simulink model "Model"  (R2019a)
settings: Solver=ode45  StartTime=0.0  StopTime=10  MaxStep=1e-3  RelTol=1e-3  EnableMultiTasking=on
values from neighbouring files (symbols this model uses):
  Cpf1 = tf(1,[1/1.05,1])    [mainProjetCADV_2a.m]
  dPHRTrim = trimVal(1)    [mainProjetCADV_2a.m]
  dthrIdle = 0.1    [mainProjetCADV_2a.m]
  H = -inv(Ccm*inv(Acm-Bcm*Kcm)*Bcm)    [mainProjetCADV_2a.m]
  idelevator = 3    [mainProjetCADV_2a.m]
  KTS2MS = 1852 / 3600    (= 0.514444444444)    [mainProjetCADV_2a.m]
  thetaTrim = trimVal(3)    [mainProjetCADV_2a.m]
  uTrim = zeros(TOTAL_CMD, 1)    [mainProjetCADV_2a.m]
  VaTrim = utEas2Tas(Eas_KTS*KTS2MS, hTrimFL*FL2M)    [mainProjetCADV_2a.m]
  xTrim = zeros(TOTAL_SV, 1)    [mainProjetCADV_2a.m]
undefined symbols (not defined in the file or in its folder): aircraftChosen, Eas_KTS, Kd, Ki, km, Kp, Ktheta, ms
settings Model: Creator=thierry  LastModifiedBy=palotaba
settings DataIOCC: LimitDataPoints=on  SaveFormat=Array  ReturnWorkspaceOutputs=off
settings OptimizationCC: LifeSpan=inf
settings DebuggingCC: UnderspecifiedInitializationDetection=Classic  MergeDetectMultiDrivingBlocksExec=none  SolverPrmCheckMsg=warning  StateNameClashWarn=warning  SFUnexpectedBacktrackingDiag=warning  SFNoUnconditionalDefaultTransitionDiag=warning  SFExecutionAtInitializationDiag=none  ArithmeticOperatorsInVariantConditions=warning
settings HardwareCC: ProdBitPerPointer=32  ProdBitPerSizeT=32  ProdBitPerPtrDiffT=32  ProdLargestAtomicFloat=None  ProdIntDivRoundTo=Undefined  ProdEndianess=Unspecified  ProdWordSize=32  ProdHWDeviceType=32-bit Generic
settings ModelReferenceCC: PropagateSignalLabelsOutOfModel=off
settings SFSimCC: SimUseLocalCustomCode=off
settings RTWCC: RTWUseLocalCustomCode=off
settings CodeAppCC: StateflowObjectComments=on
settings GRTTargetCC: TargetLangStandard=C89/C90 (ANSI)
settings ConfigComp: CovMetricSettings=dw  CovSaveCumulativeToWorkspaceVar=on  CovSaveSingleToWorkspaceVar=on  CovExternalEMLEnable=off

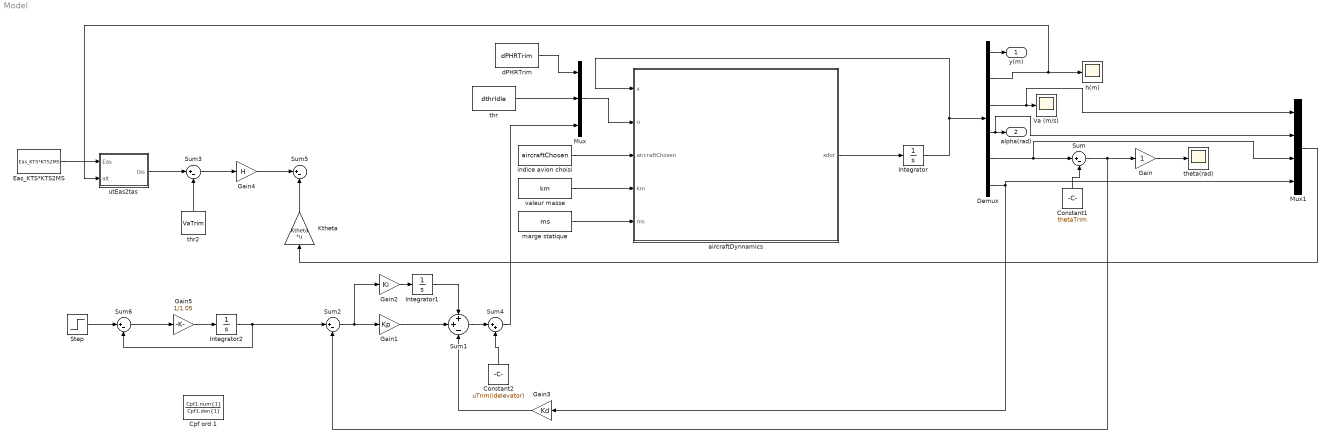
== system Model ==
  Constant1 : Constant  Value=thetaTrim
  Constant2 : Constant  Value=uTrim(idelevator)
  "Cpf ord 1 " : TransferFcn  Numerator=Cpf1.num{1}  Denominator=Cpf1.den{1}
  Demux : Demux  Outputs=6
  Eas_KTS*KTS2MS : Constant  Value=Eas_KTS*KTS2MS
  Gain : Gain
  Gain1 : Gain  Gain=Kp
  Gain2 : Gain  Gain=Ki
  Gain3 : Gain  Gain=Kd
  Gain4 : Gain  Gain=H
  Gain5 : Gain  Gain=1/1.05
  Integrator : Integrator  InitialCondition=xTrim
  Integrator1 : Integrator
  Integrator2 : Integrator
  "Ktheta " : Gain  Gain=Ktheta  Multiplication=Matrix(K*u) (u vector)
  Mux : Mux  Inputs=3
  Mux1 : Mux
  Step : Step  Time=0  After=0.1  SampleTime=0
  Sum{,2..3,5..6} (5 alike) : Sum  Inputs=|+-
  Sum1 : Sum  Inputs=++-
  Sum4 : Sum  Inputs=|++
  "Va (m/s) " : Scope
  aircraftDynnamics : MATLAB Function  TreatAsAtomicUnit=on
  dPHRTrim : Constant  Value=dPHRTrim
  h(m) : Scope
  indice avion choisi : Constant  Value=aircraftChosen
  marge statique : Constant  Value=ms
  theta(rad) : Scope
  thr : Constant  Value=dthrIdle
  thr2 : Constant  Value=VaTrim
  utEas2tas : MATLAB Function  TreatAsAtomicUnit=on
  valeur masse : Constant  Value=km
  y(m) : Outport
  alpha(rad) : Outport  Port=2
  wires:
  aircraftDynnamics/1(xdot) -> Integrator/1
  Integrator/1 -> aircraftDynnamics/1(x), Demux/1
  valeur masse/1 -> aircraftDynnamics/4(km)
  indice avion choisi/1 -> aircraftDynnamics/3(aircraftChosen)
  marge statique/1 -> aircraftDynnamics/5(ms)
  Mux/1 -> aircraftDynnamics/2(u)
  dPHRTrim/1 -> Mux/1
  thr/1 -> Mux/2
  Demux/1 -> y(m)/1
  Demux/4 -> Mux1/2, alpha(rad)/1
  Demux/6 -> Gain3/1, Mux1/4
  Demux/3 -> Mux1/1, "Va (m/s) "/1
  Demux/2 -> utEas2tas/2(alt), h(m)/1
  Gain/1 -> theta(rad)/1
  Integrator1/1 -> Sum1/1
  Constant1/1 -> Sum/2
  Sum/1 -> Sum2/2, Gain/1
  Gain3/1 -> Sum1/3
  Gain1/1 -> Sum1/2
  Gain2/1 -> Integrator1/1
  Sum2/1 -> Gain2/1, Gain1/1
  Demux/5 -> Mux1/3, Sum/1
  Constant2/1 -> Sum4/2
  Sum4/1 -> Mux/3
  Sum1/1 -> Sum4/1
  Eas_KTS*KTS2MS/1 -> utEas2tas/1(Eas)
  utEas2tas/1(tas) -> Sum3/1
  thr2/1 -> Sum3/2
  Sum3/1 -> Gain4/1
  "Ktheta "/1 -> Sum5/2
  Gain4/1 -> Sum5/1
  Mux1/1 -> "Ktheta "/1
  Step/1 -> Sum6/1
  Sum6/1 -> Gain5/1
  Integrator2/1 -> Sum6/2, Sum2/1
  Gain5/1 -> Integrator2/1

== matlab function Model/aircraftDynnamics ==
  data: x input; u input; xdot output; aircraftChosen input; km input; ms input
function xdot = aircraftDynamics(x,u, aircraftChosen,km,ms)
    TOTAL_SV = 6;
    xIn = zeros(TOTAL_SV,1);
    xIn = x;
    
	TOTAL_CMD = 3;
    uIn = zeros(TOTAL_CMD,1);
    uIn = u;
    
    xdot = utAcDynamicsFunction(xIn,uIn, aircraftChosen,km,ms);
end %aircraftDynamics

== matlab function Model/utEas2tas ==
  data: Eas input; tas output; alt input
function tas = utEas2tas(Eas, alt)
    %tas, Eas (%equivalent vitesse) en m/s
    %alt en m
    %cf. http://www.hochwarth.com/misc/AviationCalculator.html
    tas = sqrt(utRho(0)/utRho(alt))*Eas;
end
